simulink model "sete_um"  (R2022b)
settings: Solver=VariableStepAuto  StartTime=0.0  StopTime=10.0  RelTol=1e-3
settings Model: Creator=Admin  LastModifiedBy=Admin

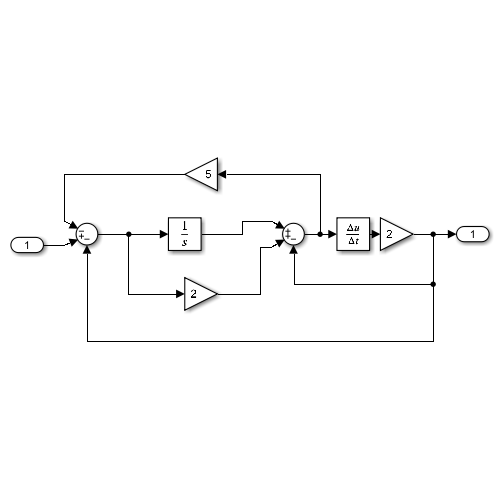
[thumbnail: Simulink's stored preview of the top-level diagram]
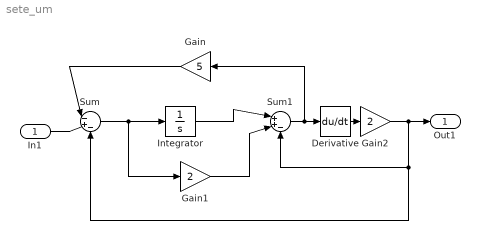
== system sete_um ==
  In1 : Inport
  Derivative : Derivative
  Gain : Gain  Gain=5
  Gain1 : Gain  Gain=2
  Gain2 : Gain  Gain=2
  Integrator : Integrator
  Sum : Sum  Inputs=|-+-
  Sum1 : Sum  Inputs=|++-
  Out1 : Outport
  wires:
  Sum1/1 -> Derivative/1, Gain/1
  Gain/1 -> Sum/1
  Gain1/1 -> Sum1/2
  Integrator/1 -> Sum1/1
  In1/1 -> Sum/2
  Gain2/1 -> Sum1/3, Sum/3, Out1/1
  Sum/1 -> Integrator/1, Gain1/1
  Derivative/1 -> Gain2/1
